simulink model "MinimalExample"  (R2016b)
settings: Solver=FixedStepDiscrete  StartTime=0.0  StopTime=inf  FixedStep=0.02  RelTol=1e-3  EnableMultiTasking=on
libraries: PaPILibrary x1
settings Model: Creator=salchow  LastModifiedBy=valtin
settings DataIOCC: LimitDataPoints=on  SaveFormat=Array
settings OptimizationCC: LifeSpan=Inf
settings DebuggingCC: SolverPrmCheckMsg=warning  SFUnexpectedBacktrackingDiag=warning  SFNoUnconditionalDefaultTransitionDiag=warning  SFExecutionAtInitializationDiag=none
settings HardwareCC: ProdBitPerPointer=32  ProdBitPerSizeT=32  ProdBitPerPtrDiffT=32  ProdLargestAtomicFloat=None  ProdIntDivRoundTo=Undefined  ProdEndianess=Unspecified  ProdWordSize=32  ProdHWDeviceType=32-bit Generic
settings ModelReferenceCC: PropagateSignalLabelsOutOfModel=off
settings RTWCC: SystemTargetFile=ert_linux.tlc  MakeCommand="make_rtw  OPTS=\"-DWITH_HW -g\""  TemplateMakefile=ert_linux.tmf  Description=Linux Embedded Coder  TargetLang=C++
settings CodeAppCC: IgnoreCustomStorageClasses=off
settings STFCustomTargetCC: ModelReferenceCompliant=off  CombineOutputUpdateFcns=on  ERTCustomFileBanners=on  SupportContinuousTime=off  SupportNonInlinedSFcns=off  RemoveResetFunc=on  MATLABClassNameForMDSCustomization=Simulink.SoftwareTarget.ERTCustomization  GRTInterface=off  SystemTargetFile=ert_linux.tlc
settings ERTTargetCC: ModelReferenceCompliant=off  ParMdlRefBuildCompliant=off  CompOptLevelCompliant=off  ConcurrentExecutionCompliant=off  ERTFirstTimeCompliant=off  ModelStepFunctionPrototypeControlCompliant=off  CPPClassGenCompliant=off  UseToolchainInfoCompliant=off  ExtMode=on  ERTCustomFileTemplate=ert_linux_file_process.tlc  ConvertIfToSwitch=off  SuppressUnreachableDefaultCases=off
settings ConfigComp: CovMetricSettings=dw  CovHtmlReporting=on  CovSaveCumulativeToWorkspaceVar=on  CovSaveSingleToWorkspaceVar=on  CovExternalEMLEnable=off  CovSFcnEnable=off

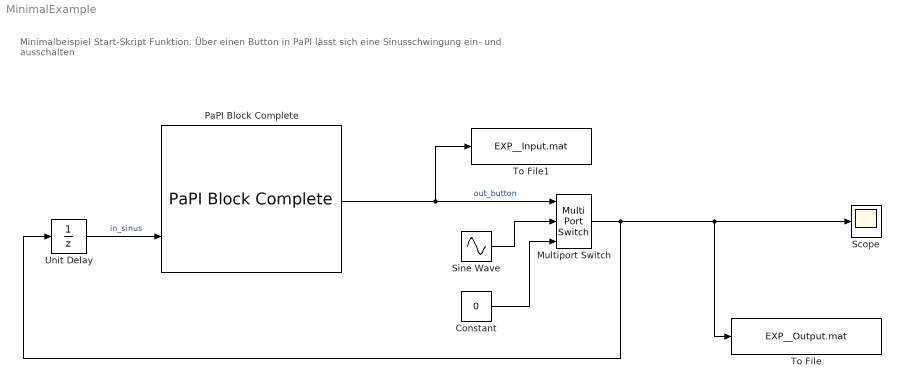
== system MinimalExample ==
  note: Minimalbeispiel Start-Skript
      | Funktion: Über einen Button in PaPI lässt sich eine Sinusschwingung ein- und ausschalten
  Constant : Constant  Value=0  SampleTime=0.02
  Multiport Switch : MultiPortSwitch  DataPortOrder=Zero-based contiguous  Inputs=2
  PaPI Block Complete : PaPILibrary/PaPI Block Complete  amount_parameters=[1]  define_inputs=[1]  split_inputs=[0]  json_string='PaPI_MinimalExample.json'  UDPLocalPort=20001  UDPRemotePort=20000  UDPRemoteIP='127.0.0.1'  UDPStart=on  SampleTime=0.02
  Scope : Scope
  Sine Wave : Sin  SineType=Sample based  Amplitude=5  Frequency=10  Samples=25  SampleTime=0.02
  To File : ToFile  Filename=EXP__Output.mat  MatrixName=output
  To File1 : ToFile  Filename=EXP__Input.mat  MatrixName=input
  Unit Delay : UnitDelay  SampleTime=-1
  wires:
  Sine Wave/1 -> Multiport Switch/2
  Constant/1 -> Multiport Switch/3
  PaPI Block Complete/1 -> To File1/1, Multiport Switch/1  "out_button"
  Multiport Switch/1 -> Unit Delay/1, To File/1, Scope/1
  Unit Delay/1 -> PaPI Block Complete/2  "in_sinus"
